simulink library "tqd"  (R2021b)
settings: Solver=VariableStepAuto  StartTime=0.0  StopTime=10.0  RelTol=1e-3
undefined symbols (not defined in the file or in its folder): ATQD_APSDecReq_X_kph, ATQD_APSDecReq_Y_mps2, ATQD_APSDecReqCMD_X_kph, ATQD_APSDecReqTs_X_pct, ATQD_APSDecTimeGain_X_Deg, ATQD_APSDecTimeGain_Y_s, ATQD_APSReqLowSpd_X_Deg, ATQD_AutoHoldReleaseBPS_X_Deg, ATQD_AWDLoadTrqnsGain_X_kg, ATQD_AWDLoadTrqnsGain_Y_pct, ATQD_BOSEnBPSPosn_X_kph, ATQD_BOSMap_X_rpm, ATQD_BOSMap_Y_pct, ATQD_CreepBaseTqD_X_kph, ATQD_CreepBaseTqD_Y_Deg, ATQD_CreepBaseTqR_X_kph, ATQD_CreepBaseTqR_Y_Deg, ATQD_CreepBPSDisPosn_X_Deg, ATQD_CreepBPSDisPosnR_X_Deg, ATQD_CreepBPSEnPosn_X_Deg, ATQD_CreepBPSEnPosnR_X_Deg, ATQD_CreepDeltaTq_X_kph, ATQD_CreepIterm_X_kph, ATQD_CreepIterm_Y_kph, ATQD_CreepItermMaxLimit_X_pct, ATQD_CreepPreloadTime_X_kph, ATQD_CreepPreloadTq_X_kph, ATQD_CreepPreloadTq_Y_s, ATQD_CreepProtTq_X_Deg, ATQD_CreepPterm_X_kph, ATQD_ECOTqMapD_X_rpm, ATQD_ECOTqMapD_Y_pct, ATQD_EOPDTqMapDCon_X_rpm, ATQD_EOPDTqMapDCon_Y_Deg, ATQD_EstInitVehWeight_X_c, ATQD_LHMRollGenMapD_X_rpm, ATQD_LHMRollGenMapD_Y_rpm, ATQD_LHMTqMapD_X_rpm, ATQD_LHMTqMapD_Y_pct, ATQD_NL1TqMapD_X_rpm, ATQD_NL1TqMapD_Y_pct, ATQD_NOPDTqMapDCon_X_rpm, ATQD_NOPDTqMapDCon_Y_Deg, ATQD_NRMRrEDUSpRat_X_rpm, ATQD_NRMRrEDUSpRat_Y_Nm, ATQD_OPDHoldDownRelDelay_X_Deg, ATQD_OPDHoldEnSpd_X_Deg, ATQD_OPDHoldRelDetTime_X_Deg, ATQD_OPDHoldReleaseTq_X_Deg, ATQD_OrigPedTqLowLim_X_Deg, ATQD_OrigPedTqLowLim_Y_pct, ATQD_PedalMapClimbUpLim_X_rpm, ATQD_PedalMapClimbUpLim_Y_Deg, ATQD_PreLoadTq_X_s, ATQD_RollGenMapEL1_X_rpm, ATQD_RollGenMapEL1_Y_rpm, ATQD_SL1TqMapD_X_rpm, ATQD_SL1TqMapD_Y_pct, ATQD_SlideRegenTqGain_X_Gps, ATQD_SlideRegenTqGain_Y_pct ... (+444)
libraries: hcu_lib x70, simulink x61, tqr x1
(part 8 of 14)

== system tqd/TQD/TorqueDemand/ShiftModule/GearShiftPosn/Drive Protection ==
  VINP_ShifterHandleCmd_enum : Inport
  VTQD_GearActualPosn_enum : Inport  Port=2
  VINP_VehSpeed_kph : Inport  Port=3
  VTQD_AfterAvailableTqDemFr_Nm : Inport  Port=4
  VTQR_NoABSREDUWhlTqReq_Nm : Inport  Port=5
  VTQR_NoABSFEDUWhlTqReq_Nm : Inport  Port=6
  VTQD_AfterAvailableTqDemRr_Nm : Inport  Port=7
  task_time_s : Inport  Port=8
  VTQD_BrkSwSta_flg : Inport  Port=9
  AND : Logic  Inputs=6  AllPortsSameDT=off  OutDataTypeStr=boolean
  AND1 : Logic  Commented=on  AllPortsSameDT=off  OutDataTypeStr=boolean
  AND2 : Logic  Inputs=3  AllPortsSameDT=off  OutDataTypeStr=boolean
  AND3 : Logic  Commented=on  Inputs=3  AllPortsSameDT=off  OutDataTypeStr=boolean
  AND4 : Logic  AllPortsSameDT=off  OutDataTypeStr=boolean
  Abs{,1,3..4} (4 alike) : Abs
  Add : Sum  Commented=on
  Add3 : Sum  Commented=on  Inputs=+++
  Constant1 : Constant  Commented=on  Value=ENUM_SHIFTCOMMAND_N
  Constant{3,6..7,10} (4 alike) : Constant  Value=KTQD_DrivProtEnToNTq_Nm
  Constant11 : Constant  Commented=on  Value=KTQD_CreepDisableSpdofst_kph
  Constant12 : Constant  Value=ENUM_SHIFTCOMMAND_N
  Constant13 : Constant  Value=KTQD_DriveProtVehSpdGain_kph
  Constant14 : Constant  Value=KTQD_DriveProtVehSpdGain_kph
  Constant16 : Constant  Value=KTQD_DrivProtEnSW_flg
  Constant17 : Constant  Value=KTQD_DriveProtDetTime_s
  Constant2 : Constant  Commented=on  Value=KTQD_DriveProtVehSpdGain_kph
  Constant20 : Constant  Commented=on  Value=ZERO_INT
  Constant21 : Constant  Commented=on  Value=ENUM_SHIFTCOMMAND_N
  Constant22 : Constant  Commented=on  Value=ENUM_SHIFTCOMMAND_N
  Constant23 : Constant  Commented=on  Value=ONE_INT
  Constant24 : Constant  Commented=on  Value=ZERO_INT
  Constant25 : Constant  Commented=on  Value=ENUM_SHIFTCOMMAND_NONE
  Constant26 : Constant  Commented=on  Value=KTQD_DriceProtDetTime_s
  Constant27 : Constant  Commented=on  Value=ENUM_SHIFTCOMMAND_D
  Constant29 : Constant  Commented=on  Value=ONE_INT
  Constant4 : Constant  Value=ENUM_GEARACTUALPOSN_D
  Constant5 : Constant  Commented=on  Value=ENUM_SHIFTCOMMAND_NONE
  Constant8 : Constant  Commented=on  Value=KTQD_DriveProtUpCount_c
  Constant9 : Constant  Commented=on  Value=KTQD_CreepEnableSpd_kph
  Delay : Delay  Commented=on  DelayLength=1
  Delay1 : Delay  Commented=on  DelayLength=1
  Delay2 : Delay  Commented=on  DelayLength=1
  Delay{4..8} (5 alike) : Delay  DelayLength=1
  DelayEnable : hcu_lib/Basic_Blocks/DelayEnable
  Detect Increase1 : simulink/Logic and Bit Operations/Detect Increase  Commented=on  vinit=0.0  OutDataTypeStr=boolean
  Equal{,2,6..7} (4 alike) : RelationalOperator  Operator=<=  OutDataTypeStr=boolean  RndMeth=Simplest
  Equal{1,4,12,15..16} (5 alike) : RelationalOperator  Commented=on  Operator===  OutDataTypeStr=boolean  RndMeth=Simplest
  Equal13 : RelationalOperator  Commented=on  Operator=~=  OutDataTypeStr=boolean  RndMeth=Simplest
  Equal14 : RelationalOperator  Commented=on  Operator=~=  OutDataTypeStr=boolean  RndMeth=Simplest
  Equal3 : RelationalOperator  Operator===  OutDataTypeStr=boolean  RndMeth=Simplest
  Equal5 : RelationalOperator  Commented=on  Operator=~=  OutDataTypeStr=boolean  RndMeth=Simplest
  Equal8 : RelationalOperator  Operator===  OutDataTypeStr=boolean  RndMeth=Simplest
  From1 : From  Commented=on  GotoTag=VINP_VehSpeed_kph
  From11 : From  Commented=on  GotoTag=VTQD_DriveProtCount_c
  From13 : From  Commented=on  GotoTag=VTQD_DriveProtDetFinish_flg
  From2 : From  Commented=on  GotoTag=VTQD_GearActualPosn_enum
  From32 : From  Commented=on  GotoTag=VTQD_DriveProtCount_c
  From{7,33..34,36} (4 alike) : From  Commented=on  GotoTag=VINP_ShifterHandleCmd_enum
  From35 : From  Commented=on  GotoTag=VTQD_DrivePortCountReset_flg
  From37 : From  Commented=on  GotoTag=VTQD_DriveProtDetFinish_flg
  From38 : From  Commented=on  GotoTag=VTQD_DriveProtDetFinish_flg
  From39 : From  Commented=on  GotoTag=task_time_s
  From40 : From  Commented=on  GotoTag=VTQD_GearActualPosn_enum
  Goto15 : Goto  Commented=on  GotoTag=VTQD_DrivePortCountReset_flg
  Goto16 : Goto  Commented=on  GotoTag=VTQD_DriveProtCount_c
  Goto17 : Goto  Commented=on  GotoTag=VTQD_DriveProtDetFinish_flg
  Goto9 : Goto  Commented=on  GotoTag=VTQD_DriveProtRemove_flg
  NOT : Logic  Commented=on  Operator=NOT  AllPortsSameDT=off  OutDataTypeStr=boolean
  NOT1 : Logic  Operator=NOT  AllPortsSameDT=off  OutDataTypeStr=boolean
  OR : Logic  Commented=on  Operator=OR  AllPortsSameDT=off  OutDataTypeStr=boolean
  OR1 : Logic  Operator=OR  AllPortsSameDT=off  OutDataTypeStr=boolean
  OR4 : Logic  Commented=on  Operator=OR  AllPortsSameDT=off  OutDataTypeStr=boolean
  OR5 : Logic  Commented=on  AllPortsSameDT=off  OutDataTypeStr=boolean
  Relational Operator1 : RelationalOperator  Commented=on  Operator=>  OutDataTypeStr=boolean  RndMeth=Simplest
  Relational Operator2 : RelationalOperator  Commented=on  OutDataTypeStr=boolean  RndMeth=Simplest
  Relational Operator3 : RelationalOperator  Operator=>  OutDataTypeStr=boolean  RndMeth=Simplest
  Relational Operator4 : RelationalOperator  Operator=<=  OutDataTypeStr=boolean  RndMeth=Simplest
  SR_Latch1 : hcu_lib/Basic_Blocks/SR_Latch  Commented=on
  SR_Latch2 : hcu_lib/Basic_Blocks/SR_Latch  Commented=on
  Switch10 : Switch  Commented=on  Criteria=u2 > Threshold
  Switch9 : Switch  Commented=on  Criteria=u2 > Threshold
  Timer : hcu_lib/Basic_Blocks/Timer  Commented=on
  VTQD_DriveProtRemove_flg : Outport
  VTQD_DriveProtToPsnN_flg : Outport  Port=2
  VTQD_DriveProtEn_flg : Outport  Port=3
  wires:
  [VTQD_DriveProtRemove_flg] -> AND/1
  Delay8/1 -> Equal3/1
  Abs4/1 -> Equal7/1
  Abs3/1 -> Equal6/1
  [VTQD_GearActualPosn_enum] -> Delay8/1
  Abs1/1 -> Equal2/1
  Abs/1 -> Equal/1
  AND2/1 -> VTQD_DriveProtEn_flg/1, DelayEnable/1  "VTQD_DriveProtEn_flg"
  Constant3/1 -> Equal/2
  Constant10/1 -> Equal2/2
  Constant6/1 -> Equal6/2
  Constant7/1 -> Equal7/2
  DelayEnable/1 -> [VTQD_DriveProtRemove_flg]  "VTQD_DriveProtRemove_flg"
  [task_time_s] -> DelayEnable/3
  Constant17/1 -> DelayEnable/2
  Constant16/1 -> AND2/2
  Equal8/1 -> AND2/1
  [VINP_VehSpeed_kph] -> Relational Operator3/1
  Constant14/1 -> Relational Operator3/2
  Constant12/1 -> Equal8/2
  [VINP_ShifterHandleCmd_enum] -> Equal8/1
  AND/1 -> [VTQD_DriveProtToPsnN_flg]  "VTQD_DriveProtToPsnN_flg"
  Delay7/1 -> [VTQD_AfterAvailableTqDemFr_Nm]
  Delay6/1 -> [VTQR_NoABSREDUWhlTqReq_Nm]
  Delay5/1 -> [VTQR_NoABSFEDUWhlTqReq_Nm]
  VTQR_NoABSFEDUWhlTqReq_Nm/1 -> Delay5/1
  Delay4/1 -> [VTQD_AfterAvailableTqDemRr_Nm]
  SR_Latch2/1 -> Goto9/1  "VTQD_DriveProtRemove_flg"
  task_time_s/1 -> [task_time_s]
  Constant2/1 -> Add3/1
  Constant11/1 -> Add3/3
  Add3/1 -> Relational Operator1/2
  Constant9/1 -> Add3/2
  VTQD_AfterAvailableTqDemRr_Nm/1 -> Delay4/1
  Equal7/1 -> AND/6
  [VTQD_AfterAvailableTqDemFr_Nm] -> Abs4/1
  Equal6/1 -> AND/5
  [VTQR_NoABSFEDUWhlTqReq_Nm] -> Abs3/1
  [VTQD_DriveProtToPsnN_flg] -> VTQD_DriveProtToPsnN_flg/1
  VTQR_NoABSREDUWhlTqReq_Nm/1 -> Delay6/1
  VTQD_AfterAvailableTqDemFr_Nm/1 -> Delay7/1
  VINP_VehSpeed_kph/1 -> [VINP_VehSpeed_kph]
  VTQD_GearActualPosn_enum/1 -> [VTQD_GearActualPosn_enum]
  VINP_ShifterHandleCmd_enum/1 -> [VINP_ShifterHandleCmd_enum]
  OR/1 -> SR_Latch2/2
  Equal5/1 -> OR/2
  Equal1/1 -> OR/1
  Constant5/1 -> Equal5/2
  From7/1 -> Equal5/1
  Constant4/1 -> Equal3/2
  Equal3/1 -> AND/4
  [VTQR_NoABSREDUWhlTqReq_Nm] -> Abs1/1
  Equal2/1 -> AND/3
  Equal/1 -> AND/2
  [VTQD_AfterAvailableTqDemRr_Nm] -> Abs/1
  [VTQD_DriveProtRemove_flg] -> VTQD_DriveProtRemove_flg/1
  Constant1/1 -> Equal1/2
  From2/1 -> Equal1/1
  Relational Operator1/1 -> AND3/3
  From1/1 -> Relational Operator1/1
  From11/1 -> Equal4/1
  From13/1 -> AND1/2
  Constant8/1 -> Equal4/2
  AND1/1 -> SR_Latch2/1  "VTQD_DriveProtEn_flg"
  Equal4/1 -> AND1/1
  Delay2/1 -> SR_Latch1/2
  Equal13/1 -> OR5/1
  Switch9/1 -> Add/1
  Switch10/1 -> Delay/1
  Constant24/1 -> Switch10/1
  From35/1 -> Switch10/2
  Detect Increase1/1 -> Switch9/2  "VTQD_ShiftNRiseDet_flg"
  From36/1 -> Equal12/1
  OR4/1 -> Goto15/1  "VTQD_DrivePortCountReset_flg"
  Equal14/1 -> OR5/2
  Add/1 -> Switch10/3
  From33/1 -> Equal13/1
  Constant29/1 -> Equal16/2
  Constant22/1 -> Equal13/2
  Delay/1 -> Add/2, Goto16/1  "VTQD_DriveProtCount_c"
  Equal15/1 -> AND3/2
  From34/1 -> Equal14/1
  Relational Operator2/1 -> Goto17/1  "VTQD_DriveProtDetFinish_flg"
  Constant20/1 -> Switch9/3
  Timer/1 -> Relational Operator2/1  "VTQD_DriveProtDetTime_s"
  OR5/1 -> OR4/2
  AND3/1 -> SR_Latch1/1  "VTQD_DriveProtTimerEn_flg"
  NOT/1 -> Timer/2
  Constant21/1 -> Equal12/2
  Constant25/1 -> Equal14/2
  From39/1 -> Timer/3
  From32/1 -> Equal16/1
  From37/1 -> Delay1/1
  From40/1 -> Equal15/1
  From38/1 -> Delay2/1
  Delay1/1 -> OR4/1
  SR_Latch1/1 -> Timer/1, NOT/1
  Constant27/1 -> Equal15/2
  Constant23/1 -> Switch9/1
  Equal16/1 -> AND3/1
  Equal12/1 -> Detect Increase1/1
  Constant26/1 -> Timer/4, Relational Operator2/2
  OR1/1 -> AND2/3
  Relational Operator3/1 -> OR1/1
  Constant13/1 -> Relational Operator4/2
  [VINP_VehSpeed_kph] -> Relational Operator4/1
  Relational Operator4/1 -> AND4/1
  AND4/1 -> OR1/2
  [VTQD_BrkSwSta_flg] -> NOT1/1
  NOT1/1 -> AND4/2
  VTQD_BrkSwSta_flg/1 -> [VTQD_BrkSwSta_flg]

== system tqd/TQD/TorqueDemand/Signal_convert/Regen Level Switch Botton/RegenDOWN ==
  note: IF PRESS BOTH then nothing happen
  note: Long press or Short press
  note: If press time more then Long press's limit then go Long press only. Else go short press only. Else if no press.
  note: IF PRESS BOTH then nothing happen
  task_time_s : Inport
  SWC_RegenUp : Inport  Port=2
  SWC_RegenDOWN : Inport  Port=3
  AND : Logic  AllPortsSameDT=off  OutDataTypeStr=boolean
  AND1 : Logic  AllPortsSameDT=off  OutDataTypeStr=boolean
  AND2 : Logic  AllPortsSameDT=off  OutDataTypeStr=boolean
  Constant{1..2,4,7,10} (5 alike) : Constant  Value=FALSE
  Constant3 : Constant  Value=KTQD_RegShortPLim_s
  Default 3 sec : Constant  Value=KTQD_RegLongPLim_s
  DelayEnable_LONG_PRESS : hcu_lib/Basic_Blocks/DelayEnable
  DelayEnable_SHORT_PRESS : hcu_lib/Basic_Blocks/DelayEnable
  Detect Decrease1 : simulink/Logic and Bit Operations/Detect Decrease  vinit=0.0  OutDataTypeStr=boolean
  Detect Decrease2 : simulink/Logic and Bit Operations/Detect Decrease  vinit=0.0  OutDataTypeStr=boolean
  Detect Increase : simulink/Logic and Bit Operations/Detect Increase  vinit=0.0  OutDataTypeStr=boolean
  NOT : Logic  Operator=NOT  AllPortsSameDT=off  OutDataTypeStr=boolean
  NOT1 : Logic  Operator=NOT  AllPortsSameDT=off  OutDataTypeStr=boolean
  SR_Latch : hcu_lib/Basic_Blocks/SR_Latch
  Switch{1..5} (5 alike) : Switch  Criteria=u2 ~= 0
  SWC_RegenDownShort_flg : Outport
  VTQD_RegenDownLongP_flg : Outport  Port=2
  wires:
  Detect Decrease1/1 -> AND/2
  SR_Latch/1 -> [PRESS_BOTH]
  AND2/1 -> SR_Latch/2
  NOT1/1 -> AND2/2
  NOT/1 -> AND2/1
  [SWC_RegenDOWN] -> NOT1/1
  [SWC_RegenUp] -> NOT/1
  Constant4/1 -> Switch5/1
  [PRESS_BOTH] -> Switch5/2
  [SWC_RegenDOWN] -> Switch5/3
  Switch4/1 -> [Short_press_falling_Edge]
  Detect Decrease2/1 -> Switch4/3
  [PRESS_BOTH] -> Switch4/2
  Constant2/1 -> Switch4/1
  Constant1/1 -> Switch3/1
  AND1/1 -> SR_Latch/1
  [SWC_RegenUp] -> AND1/1
  [SWC_RegenDOWN] -> AND1/2
  [PRESS_BOTH] -> Switch3/2
  SWC_RegenDOWN/1 -> [SWC_RegenDOWN]
  SWC_RegenUp/1 -> [SWC_RegenUp]
  Switch3/1 -> [Long_press]
  Switch2/1 -> SWC_RegenDownShort_flg/1
  AND/1 -> Switch2/2
  Switch5/1 -> DelayEnable_LONG_PRESS/1, DelayEnable_SHORT_PRESS/1
  [Short_press_falling_Edge] -> Switch2/3
  Constant10/1 -> Switch2/1
  [Long_press] -> Detect Increase/1, Detect Decrease1/1
  [Short_press_falling_Edge] -> AND/1
  Switch1/1 -> Switch3/3
  DelayEnable_LONG_PRESS/1 -> Switch1/2, Switch1/1
  Constant7/1 -> Switch1/3
  DelayEnable_SHORT_PRESS/1 -> Detect Decrease2/1
  Constant3/1 -> DelayEnable_SHORT_PRESS/2
  [task_time_s] -> DelayEnable_SHORT_PRESS/3
  Default 3 sec/1 -> DelayEnable_LONG_PRESS/2
  [task_time_s] -> DelayEnable_LONG_PRESS/3
  Detect Increase/1 -> VTQD_RegenDownLongP_flg/1
  task_time_s/1 -> [task_time_s]

== system tqd/TQD/TorqueDemand/Signal_convert/Regen Level Switch Botton/RegenUP ==
  note: IF PRESS BOTH then nothing happen
  note: Long press or Short press
  note: If press time more then Long press's limit then go Long press only. Else go short press only. Else if no press.
  note: IF PRESS BOTH then nothing happen
  task_time_s : Inport
  SWC_RegenUp : Inport  Port=2
  SWC_RegenDOWN : Inport  Port=3
  AND : Logic  AllPortsSameDT=off  OutDataTypeStr=boolean
  AND1 : Logic  AllPortsSameDT=off  OutDataTypeStr=boolean
  AND2 : Logic  AllPortsSameDT=off  OutDataTypeStr=boolean
  Constant{1..2,4,7,10} (5 alike) : Constant  Value=FALSE
  Constant3 : Constant  Value=KTQD_RegShortPLim_s
  Default 3 sec : Constant  Value=KTQD_RegLongPLim_s
  DelayEnable_LONG_PRESS : hcu_lib/Basic_Blocks/DelayEnable
  DelayEnable_SHORT_PRESS : hcu_lib/Basic_Blocks/DelayEnable
  Detect Decrease1 : simulink/Logic and Bit Operations/Detect Decrease  vinit=0.0  OutDataTypeStr=boolean
  Detect Decrease2 : simulink/Logic and Bit Operations/Detect Decrease  vinit=0.0  OutDataTypeStr=boolean
  Detect Increase : simulink/Logic and Bit Operations/Detect Increase  vinit=0.0  OutDataTypeStr=boolean
  NOT : Logic  Operator=NOT  AllPortsSameDT=off  OutDataTypeStr=boolean
  NOT1 : Logic  Operator=NOT  AllPortsSameDT=off  OutDataTypeStr=boolean
  SR_Latch : hcu_lib/Basic_Blocks/SR_Latch
  Switch{1..5} (5 alike) : Switch  Criteria=u2 ~= 0
  SWC_RegenUpShort_flg : Outport
  VTQD_RegenUpLongP_flg : Outport  Port=2
  wires:
  Detect Decrease1/1 -> AND/2
  SR_Latch/1 -> [PRESS_BOTH]
  AND2/1 -> SR_Latch/2
  NOT1/1 -> AND2/2
  NOT/1 -> AND2/1
  [SWC_RegenDOWN] -> NOT1/1
  [SWC_RegenUp] -> NOT/1
  Constant4/1 -> Switch5/1
  [PRESS_BOTH] -> Switch5/2
  [SWC_RegenUp] -> Switch5/3
  Switch4/1 -> [Short_press_falling_Edge]
  Detect Decrease2/1 -> Switch4/3
  [PRESS_BOTH] -> Switch4/2
  Constant2/1 -> Switch4/1
  Constant1/1 -> Switch3/1
  AND1/1 -> SR_Latch/1
  [SWC_RegenUp] -> AND1/1
  [SWC_RegenDOWN] -> AND1/2
  [PRESS_BOTH] -> Switch3/2
  SWC_RegenDOWN/1 -> [SWC_RegenDOWN]
  SWC_RegenUp/1 -> [SWC_RegenUp]
  Switch3/1 -> [Long_press]
  Switch2/1 -> SWC_RegenUpShort_flg/1
  AND/1 -> Switch2/2
  Switch5/1 -> DelayEnable_LONG_PRESS/1, DelayEnable_SHORT_PRESS/1
  [Short_press_falling_Edge] -> Switch2/3
  Constant10/1 -> Switch2/1
  [Long_press] -> Detect Increase/1, Detect Decrease1/1
  [Short_press_falling_Edge] -> AND/1
  Switch1/1 -> Switch3/3
  DelayEnable_LONG_PRESS/1 -> Switch1/2, Switch1/1
  Constant7/1 -> Switch1/3
  DelayEnable_SHORT_PRESS/1 -> Detect Decrease2/1
  Constant3/1 -> DelayEnable_SHORT_PRESS/2
  [task_time_s] -> DelayEnable_SHORT_PRESS/3
  Default 3 sec/1 -> DelayEnable_LONG_PRESS/2
  [task_time_s] -> DelayEnable_LONG_PRESS/3
  Detect Increase/1 -> VTQD_RegenUpLongP_flg/1
  task_time_s/1 -> [task_time_s]

== system tqd/TQD/TorqueDemand/Signal_convert/Speed Setting Mode/ACC Speed Setting ON ==
  note: ACC SPEED SETTING MODE
  VTQD_SWCResUpSta_flg : Inport
  VTQD_SWCSetDownSta_flg : Inport  Port=2
  task_time_s : Inport  Port=3
  VVMC_LVDAACCStatusInformation_flg : Inport  Port=4
  VVMC_ACCObjDist_m : Inport  Port=5
  VVMC_MeterIndSpeed_raw32 : Inport  Port=6
  VINP_ADASACCSta_enum : Inport  Port=7
  VINP_Distanceunit_flg : Inport  Port=8
  Action Port : ActionPort  InitializeStates=reset
  " 20" : Constant  Value=KTQD_ACCActiveMetSpdLoMPH_mph
  " 30kph" : Constant  Value=KTQD_ACCActiveMetSpdLo_kph
  0 : Constant  Value=KTQD_AllowSetSpdOvrd_flg
  1 : Constant  Value=KTQD_AllowSetSpdOvrdVal_flg
  1.1s : Constant  Value=KTQD_SetSpdLongPLim_s
  105 : Constant  Value=KTQD_ACCActiveMetSpdHiMPH_mph
  10kph1 : Constant  Value=KTQD_AllowSetSpdSpd_kph
  180kph : Constant  Value=KTQD_ACCActiveMetSpdHi_kph
  20m : Constant  Value=KTQD_AllowSetSpdDist_m
  2m : Constant  Value=KTQD_NotAllowSetSpdDist_m
  5 : Constant  Value=KTQD_SetSpdDeltaLongMPH_mph
  5kph : Constant  Value=KTQD_SetSpdDeltaLong_kph
  ACCSetSpd_Chart_W : Stateflow chart  TreatAsAtomicUnit=on
      settings: PortSchema="{\"entries\":[{\"content\":{\"sides\":[{\"content\":{\"connectorIds\":[\"In1\",\"In2\",\"In3\",\"In4\",\"In5\",\"In6\",\"In7\",\"In8\",\"In12\",\"In9\",\"In10\",\"In11\"]},\"type\":\"ConnectorPlacement.EquallySpacedRectSide\",\"uuid\":\"61ce72b2-2f56-4065-9e06-1345412a8c86\"},{\"content\":{\"connectorIds\":[\"Out1\"],\"side\":\"RIGHT\"},\"type\":\"ConnectorPlacement.EquallySpacedRectSide\",\"uuid\":\"4594d6d3-f7cd-4711-8df0-9a0a2c5601b5\"},{\"content\":{\"connectorIds\":[],\"side\":\"TOP\"},\"type\":\"ConnectorPlacement.EquallySpacedRectSide\",\"uuid\":\"a8857ab2-f9b0-4737-b2f3-522f42c1ada3\"}]},\"type\":\"ConnectorPlacement.EquallySpacedConnector\",\"uuid\":\"0a7f8e6a-9c19-454d-bd26-d3d8923cc49e\"}],\"packageUris\":[\"http://schema.mathworks.com/mf0/Connector/R2020b\"],\"version\":\"1.0\"}"
  AND : Logic  AllPortsSameDT=off  OutDataTypeStr=boolean
  AND1 : Logic  AllPortsSameDT=off  OutDataTypeStr=boolean
  Cast To Single : DataTypeConversion  OutDataTypeStr=int8
  ONE : Constant  Value=ONE_INT
  OR : Logic  Operator=OR  AllPortsSameDT=off  OutDataTypeStr=boolean
  Relational Operator : RelationalOperator  Operator=<=  OutDataTypeStr=boolean  RndMeth=Simplest
  Relational Operator1 : RelationalOperator  Operator=>  OutDataTypeStr=boolean  RndMeth=Simplest
  Relational Operator2 : RelationalOperator  Operator===  OutDataTypeStr=boolean  RndMeth=Simplest
  Relational Operator3 : RelationalOperator  OutDataTypeStr=boolean  RndMeth=Simplest
  Relational Operator4 : RelationalOperator  Operator===  OutDataTypeStr=boolean  RndMeth=Simplest
  Round : Rounding  Operator=round
  Switch{,1..4} (5 alike) : Switch  Criteria=u2 > Threshold
  standby : Constant  Value=ENUM_ADASACCSTA_STANDBY
  zero : Constant  Value=ZERO_INT
  VTQD_ACCSetSpd_kph : Outport
  wires:
  VVMC_LVDAACCStatusInformation_flg/1 -> ACCSetSpd_Chart_W/10(VVMC_LVDAACCStatusInformation_flg)
  1.1s/1 -> ACCSetSpd_Chart_W/9(KTQD_SetSpdLongPLim_s)
  task_time_s/1 -> ACCSetSpd_Chart_W/12(task_time_s)
  Switch4/1 -> ACCSetSpd_Chart_W/8(KTQD_SetSpdDeltaLong_kph)
  Switch3/1 -> ACCSetSpd_Chart_W/7(KTQD_ACCActiveMetSpdLo_raw32)
  180kph/1 -> Switch2/3
  VVMC_MeterIndSpeed_raw32/1 -> ACCSetSpd_Chart_W/4(VVMC_MeterIndSpeed_raw32), [VVMC_MeterIndSpeed_raw32]
  VTQD_SWCSetDownSta_flg/1 -> ACCSetSpd_Chart_W/3(VTQD_SWCSetDownSta_flg)
  VTQD_SWCResUpSta_flg/1 -> ACCSetSpd_Chart_W/2(VTQD_SWCResUpSta_flg)
  VINP_ADASACCSta_enum/1 -> [VINP_ADASACCSta_enum], ACCSetSpd_Chart_W/1(VINP_ADASACCSta_enum)
  VVMC_ACCObjDist_m/1 -> Relational Operator/1, Relational Operator1/1
  20m/1 -> Relational Operator/2
  2m/1 -> Relational Operator1/2
  Relational Operator/1 -> AND/1
  Relational Operator1/1 -> AND/2
  [VVMC_MeterIndSpeed_raw32] -> Relational Operator3/1
  10kph1/1 -> Relational Operator3/2
  AND/1 -> OR/1
  Relational Operator3/1 -> OR/2
  Switch/1 -> [VTQD_AllowSetSpd_flg]
  OR/1 -> Switch/3
  0/1 -> Switch/2
  1/1 -> Switch/1
  [VTQD_AllowSetSpd_flg] -> ACCSetSpd_Chart_W/11(VTQD_AllowSetSpd_flg)
  Cast To Single/1 -> Relational Operator4/1, Switch1/3
  Switch1/1 -> VTQD_ACCSetSpd_kph/1
  [VINP_ADASACCSta_enum] -> Relational Operator2/1
  AND1/1 -> Switch1/2
  ONE/1 -> Switch1/1
  standby/1 -> Relational Operator2/2
  zero/1 -> Relational Operator4/2
  Relational Operator2/1 -> AND1/1
  Relational Operator4/1 -> AND1/2
  VINP_Distanceunit_flg/1 -> [VINP_Distanceunit_flg]
  [VINP_Distanceunit_flg] -> Switch2/2
  105/1 -> Switch2/1
  Switch2/1 -> ACCSetSpd_Chart_W/5(KTQD_ACCActiveMetSpdHi_raw32)
  [VINP_Distanceunit_flg] -> Switch3/2
  " 30kph"/1 -> Switch3/3
  " 20"/1 -> Switch3/1
  [VINP_Distanceunit_flg] -> Switch4/2
  5kph/1 -> Switch4/3
  5/1 -> Switch4/1
  [VINP_Distanceunit_flg] -> ACCSetSpd_Chart_W/6(VINP_Distanceunit_flg)
  Round/1 -> Cast To Single/1
  ACCSetSpd_Chart_W/1(VTQD_ACCSetSpd_kph) -> Round/1

== system tqd/TQD/TorqueDemand/Signal_convert/Speed Setting Mode/CC Speed Setting ON ==
  note: CC SPEED SETTING MODE
  VVMC_CCCtrlSta_enum : Inport
  "VTQD_SWCResUpPress_enum  " : Inport  Port=2
  "VTQD_SWCSetDownPress_enum  " : Inport  Port=3
  VVMC_MeterIndSpeed_raw32 : Inport  Port=4
  VTQD_SetSpdDeltaLongFit_kph : Inport  Port=5
  VINP_Distanceunit_flg : Inport  Port=6
  Action Port : ActionPort  InitializeStates=reset
  " 1" : Constant  Value=KTQD_CCActiveMetSpdLo_kph
  " 2" : Constant  Value=KTQD_CCActiveMetSpdLoMPH_mph
  1 : Constant  Value=KTQD_SetSpdDeltaLongFit_kph
  2 : Constant  Value=KTQD_SetSpdDeltaShort_kph
  3 : Constant  Value=KTQD_CCActiveMetSpdHi_kph
  4 : Constant  Value=KTQD_SetSpdDeltaLong_kph
  5 : Constant  Value=KTQD_CCActiveMetSpdHiMPH_mph
  6 : Constant  Value=KTQD_SetSpdDeltaLongMPH_mph
  AND1 : Logic  AllPortsSameDT=off  OutDataTypeStr=boolean
  CC Speed Setting Mode : Stateflow chart  TreatAsAtomicUnit=on
      settings: PortSchema="{\"entries\":[{\"content\":{\"sides\":[{\"content\":{\"connectorIds\":[\"In5\",\"In12\",\"In4\",\"In3\",\"In9\",\"In6\",\"In7\",\"In8\",\"In1\",\"In2\",\"In11\",\"In10\"]},\"type\":\"ConnectorPlacement.EquallySpacedRectSide\",\"uuid\":\"331c8dfa-4564-419d-9323-fdbf8561d50b\"},{\"content\":{\"connectorIds\":[\"Out1\",\"Out2\"],\"side\":\"RIGHT\"},\"type\":\"ConnectorPlacement.EquallySpacedRectSide\",\"uuid\":\"71cb1444-7708-4b6f-91dd-d8a1c8c14ea8\"},{\"content\":{\"connectorIds\":[],\"side\":\"TOP\"},\"type\":\"ConnectorPlacement.EquallySpacedRectSide\",\"uuid\":\"6ecf38bb-d171-491a-a8b2-073f135e7039\"}]},\"type\":\"ConnectorPlacement.EquallySpacedConnector\",\"uuid\":\"fc3afa97-6e6e-4933-9aff-7c8f8cbb1702\"}],\"packageUris\":[\"http://schema.mathworks.com/mf0/Connector/R2020b\"],\"version\":\"1.0\"}"
  Cast To Single : DataTypeConversion  OutDataTypeStr=int8
  ONE : Constant  Value=ONE_INT
  Relational Operator2 : RelationalOperator  Operator===  OutDataTypeStr=boolean  RndMeth=Simplest
  Relational Operator4 : RelationalOperator  Operator===  OutDataTypeStr=boolean  RndMeth=Simplest
  Round : Rounding  Operator=round
  Specific_STATE_ChangeToSTANDBY : Stateflow chart  TreatAsAtomicUnit=on
  Switch{1..4} (4 alike) : Switch  Criteria=u2 > Threshold
  Terminator1 : Terminator
  standby : Constant  Value=ENUM_ADASCCSTA_STANDBY
  zero : Constant  Value=ZERO_INT
  VTQD_CCSetSpd_kph : Outport
  wires:
  "VTQD_SWCSetDownPress_enum  "/1 -> CC Speed Setting Mode/10(VTQD_SWCSetDownPress_enum)
  [VTQD_ChangeToSTANDBY_flg] -> CC Speed Setting Mode/12(VTQD_ChangeToSTANDBY_flg)
  Specific_STATE_ChangeToSTANDBY/1(VTQD_CCChangeToSTANDBY_flg) -> [VTQD_ChangeToSTANDBY_flg]  "VTQD_CCChangeToSTANDBY_flg"
  [VVMC_CCCtrlSta_enum] -> Specific_STATE_ChangeToSTANDBY/1(VVMC_CCCtrlSta_enum)
  "VTQD_SWCResUpPress_enum  "/1 -> CC Speed Setting Mode/11(VTQD_SWCResUpPress_enum)
  VVMC_CCCtrlSta_enum/1 -> CC Speed Setting Mode/5(VVMC_CCCtrlSta_enum), [VVMC_CCCtrlSta_enum]
  Switch2/1 -> CC Speed Setting Mode/7(KTQD_CCActiveMetSpdHi_raw32)
  2/1 -> CC Speed Setting Mode/2(KTQD_SetSpdDeltaShort_kph)
  Switch3/1 -> CC Speed Setting Mode/8(KTQD_CCActiveMetSpdLo_raw32)
  Switch4/1 -> CC Speed Setting Mode/1(KTQD_SetSpdDeltaLong_kph)
  CC Speed Setting Mode/2(VTQD_CCSpdResetFinish_flg) -> Terminator1/1  "VTQD_CCSpdResetFinish_flg"
  VTQD_SetSpdDeltaLongFit_kph/1 -> CC Speed Setting Mode/4(VTQD_SetSpdDeltaLongFit_kph)
  1/1 -> CC Speed Setting Mode/3(KTQD_SetSpdDeltaLongFit_kph)
  VVMC_MeterIndSpeed_raw32/1 -> CC Speed Setting Mode/9(VVMC_MeterIndSpeed_raw32)
  Cast To Single/1 -> Relational Operator4/1, Switch1/3
  Switch1/1 -> VTQD_CCSetSpd_kph/1
  [VVMC_CCCtrlSta_enum] -> Relational Operator2/1
  AND1/1 -> Switch1/2
  ONE/1 -> Switch1/1
  standby/1 -> Relational Operator2/2
  zero/1 -> Relational Operator4/2
  Relational Operator2/1 -> AND1/1
  Relational Operator4/1 -> AND1/2
  [VINP_Distanceunit_flg] -> Switch2/2
  VINP_Distanceunit_flg/1 -> [VINP_Distanceunit_flg]
  3/1 -> Switch2/3
  5/1 -> Switch2/1
  [VINP_Distanceunit_flg] -> Switch3/2
  " 1"/1 -> Switch3/3
  " 2"/1 -> Switch3/1
  [VINP_Distanceunit_flg] -> Switch4/2
  4/1 -> Switch4/3
  6/1 -> Switch4/1
  [VINP_Distanceunit_flg] -> CC Speed Setting Mode/6(VINP_Distanceunit_flg)
  Round/1 -> Cast To Single/1
  CC Speed Setting Mode/1(VTQD_CCSetSpd_kph) -> Round/1

== system tqd/TQD/TorqueDemand/Signal_convert/Speed Setting Mode/Else Speed Setting On ==
  In : Inport
  Action Port : ActionPort
  Data Type Conversion : DataTypeConversion
  Out : Outport
  wires:
  Data Type Conversion/1 -> Out/1
  In/1 -> Data Type Conversion/1

== system tqd/TQD/TorqueDemand/Signal_convert/Speed Setting Mode/ISA Speed Setting ON ==
  VINP_ADASVehSpdLim_kph : Inport
  Action Port : ActionPort
  Data Type Conversion : DataTypeConversion
  VTQD_ISASetSpd_kph : Outport
  wires:
  VINP_ADASVehSpdLim_kph/1 -> Data Type Conversion/1
  Data Type Conversion/1 -> VTQD_ISASetSpd_kph/1

== system tqd/TQD/TorqueDemand/Signal_convert/Speed Setting Mode/MSA Speed Setting ON ==
  note: MSA SPEED SETTING MODE
  VVMC_MSACrlSta_enum : Inport
  "VTQD_SWCResUpPress_enum  " : Inport  Port=2
  "VTQD_SWCSetDownPress_enum  " : Inport  Port=3
  VVMC_MeterIndSpeed_raw32 : Inport  Port=4
  VTQD_SetSpdDeltaLongFit_kph : Inport  Port=5
  VINP_Distanceunit_flg : Inport  Port=6
  Action Port : ActionPort  InitializeStates=reset
  " 1" : Constant  Value=KTQD_MSAActiveMetSpdLoMPH_mph
  " 80" : Constant  Value=KTQD_MSAActiveMetSpdLo_kph
  1 : Constant  Value=KTQD_SetSpdDeltaShort_kph
  160 : Constant  Value=KTQD_MSAActiveMetSpdHi_kph
  2 : Constant  Value=KTQD_MSAActiveMetSpdHiMPH_mph
  3 : Constant  Value=KTQD_SetSpdDeltaLongMPH_mph
  5 : Constant  Value=KTQD_SetSpdDeltaLong_kph
  AND1 : Logic  AllPortsSameDT=off  OutDataTypeStr=boolean
  Cast To Single : DataTypeConversion  OutDataTypeStr=int8
  Delta Long Fit Base : Constant  Value=KTQD_SetSpdDeltaLongFit_kph
  MSA : Stateflow chart  TreatAsAtomicUnit=on
      settings: PortSchema="{\"entries\":[{\"content\":{\"sides\":[{\"content\":{\"connectorIds\":[\"In9\",\"In6\",\"In5\",\"In4\",\"In7\",\"In8\",\"In1\",\"In2\",\"In12\",\"In10\",\"In11\",\"In3\"]},\"type\":\"ConnectorPlacement.EquallySpacedRectSide\",\"uuid\":\"4fee65fe-2e32-4dfc-9c8c-ef7087e97952\"},{\"content\":{\"connectorIds\":[\"Out1\"],\"side\":\"RIGHT\"},\"type\":\"ConnectorPlacement.EquallySpacedRectSide\",\"uuid\":\"8d915692-cb0b-4a06-a57e-690cea51e532\"},{\"content\":{\"connectorIds\":[],\"side\":\"TOP\"},\"type\":\"ConnectorPlacement.EquallySpacedRectSide\",\"uuid\":\"3fa43362-4ddf-4693-9d82-d4f790f00c9c\"}]},\"type\":\"ConnectorPlacement.EquallySpacedConnector\",\"uuid\":\"c1a6cfdc-58f2-45b0-af62-575976a00cf2\"}],\"packageUris\":[\"http://schema.mathworks.com/mf0/Connector/R2020b\"],\"version\":\"1.0\"}"
  ONE : Constant  Value=ONE_INT
  Relational Operator2 : RelationalOperator  Operator===  OutDataTypeStr=boolean  RndMeth=Simplest
  Relational Operator4 : RelationalOperator  Operator===  OutDataTypeStr=boolean  RndMeth=Simplest
  Round : Rounding  Operator=round
  Specific_STATE_ChangeToOFF : Stateflow chart  TreatAsAtomicUnit=on
  Switch{1..4} (4 alike) : Switch  Criteria=u2 > Threshold
  standby : Constant  Value=ENUM_ADASMSASTA_STANDBY
  zero : Constant  Value=ZERO_INT
  VSCP_MSASetSpd_kph : Outport
  wires:
  VVMC_MeterIndSpeed_raw32/1 -> MSA/6(VVMC_MeterIndSpeed_raw32)
  Delta Long Fit Base/1 -> MSA/11(KTQD_SetSpdDeltaLongFit_kph)
  VTQD_SetSpdDeltaLongFit_kph/1 -> MSA/10(VTQD_SetSpdDeltaLongFit_kph)
  Switch2/1 -> MSA/7(KTQD_MSAActiveMetSpdHi_raw32)
  Switch3/1 -> MSA/8(KTQD_MSAActiveMetSpdLo_raw32)
  VVMC_MSACrlSta_enum/1 -> [VINP_MSACrlSta_enum], MSA/9(VVMC_MSACrlSta_enum)
  1/1 -> MSA/2(KTQD_SetSpdDeltaShort_kph)
  Switch4/1 -> MSA/1(KTQD_SetSpdDeltaLong_kph)
  [VTQD_ChangeToOFF_flg] -> MSA/5(VTQD_ChangeToOFF_flg)
  "VTQD_SWCSetDownPress_enum  "/1 -> MSA/3(VTQD_SWCSetDownPress_enum)
  "VTQD_SWCResUpPress_enum  "/1 -> MSA/12(VTQD_SWCResUpPress_enum)
  Specific_STATE_ChangeToOFF/1(VTQD_ChangeToOFF_flg) -> [VTQD_ChangeToOFF_flg]  "VTQD_ChangeToOFF_flg"
  [VINP_MSACrlSta_enum] -> Specific_STATE_ChangeToOFF/1(VINP_MSACrlSta_enum)
  AND1/1 -> Switch1/2
  zero/1 -> Relational Operator4/2
  standby/1 -> Relational Operator2/2
  ONE/1 -> Switch1/1
  Cast To Single/1 -> Relational Operator4/1, Switch1/3
  Relational Operator2/1 -> AND1/1
  [VINP_MSACrlSta_enum] -> Relational Operator2/1
  Relational Operator4/1 -> AND1/2
  Switch1/1 -> VSCP_MSASetSpd_kph/1
  [VINP_Distanceunit_flg] -> Switch2/2
  VINP_Distanceunit_flg/1 -> [VINP_Distanceunit_flg]
  160/1 -> Switch2/3
  2/1 -> Switch2/1
  [VINP_Distanceunit_flg] -> Switch3/2
  " 80"/1 -> Switch3/3
  " 1"/1 -> Switch3/1
  [VINP_Distanceunit_flg] -> Switch4/2
  5/1 -> Switch4/3
  3/1 -> Switch4/1
  [VINP_Distanceunit_flg] -> MSA/4(VINP_Distanceunit_flg)
  Round/1 -> Cast To Single/1
  MSA/1(VTQD_MSASetSpd_kph) -> Round/1

== system tqd/TQD/TorqueDemand/Signal_convert/Speed Setting Mode/VTQD_SWCCancelP_flg ==
  INPUT : Inport
  Detect Decrease : simulink/Logic and Bit Operations/Detect Decrease  vinit=0.0  OutDataTypeStr=boolean
  Falling_edge : Outport
  wires:
  Detect Decrease/1 -> Falling_edge/1
  INPUT/1 -> Detect Decrease/1

== system tqd/TQD/TorqueDemand/Signal_convert/Speed Setting Mode/VTQD_SWCResUpPress_enum ==
  note: Long press or Short press
  INPUT : Inport
  task_time_s : Inport  Port=2
  AND : Logic  AllPortsSameDT=off  OutDataTypeStr=boolean
  AND1 : Logic  AllPortsSameDT=off  OutDataTypeStr=boolean
  Constant2 : Constant  Value=KTQD_SetSpdShortPLim_s
  Constant3 : Constant  Value=KTQD_SetSpdLongPLim_s
  Constant4 : Constant  Value=ENUM_SWCBOTTONPRESS_LONGPRESS
  Constant5 : Constant  Value=ENUM_SWCBOTTONPRESS_SHORTPRESS
  Constant6 : Constant  Value=ENUM_SWCBOTTONPRESS_NOPRESS
  Delay : Delay  DelayLength=1
  DelayEnable_LONG_PRESS1 : hcu_lib/Basic_Blocks/DelayEnable
  DelayEnable_SHORT_PRESS1 : hcu_lib/Basic_Blocks/DelayEnable
  Detect Decrease : simulink/Logic and Bit Operations/Detect Decrease  vinit=0.0  OutDataTypeStr=boolean
  Detect Decrease4 : simulink/Logic and Bit Operations/Detect Decrease  vinit=0.0  OutDataTypeStr=boolean
  NOT : Logic  Operator=NOT  AllPortsSameDT=off  OutDataTypeStr=boolean
  NOT1 : Logic  Operator=NOT  AllPortsSameDT=off  OutDataTypeStr=boolean
  SR_Latch : hcu_lib/Basic_Blocks/SR_Latch
  Switch : Switch  Criteria=u2 ~= 0
  Switch3 : Switch  Criteria=u2 ~= 0
  OUTPUT : Outport
  wires:
  [Short_press_falling_Edge] -> Switch3/2
  Detect Decrease/1 -> SR_Latch/2
  [INPUT] -> Detect Decrease/1
  NOT1/1 -> AND1/2
  SR_Latch/1 -> NOT1/1
  [INPUT] -> AND1/1
  AND1/1 -> DelayEnable_SHORT_PRESS1/1
  [Long_press_falling_edge] -> SR_Latch/1
  [INPUT] -> AND/1
  AND/1 -> DelayEnable_LONG_PRESS1/1
  NOT/1 -> AND/2
  Delay/1 -> NOT/1
  [Long_press_falling_edge] -> Delay/1
  INPUT/1 -> [INPUT]
  task_time_s/1 -> [task_time_s]
  DelayEnable_LONG_PRESS1/1 -> [Long_press_falling_edge]
  Switch3/1 -> Switch/3
  DelayEnable_SHORT_PRESS1/1 -> Detect Decrease4/1
  Constant3/1 -> DelayEnable_LONG_PRESS1/2
  Constant2/1 -> DelayEnable_SHORT_PRESS1/2
  [task_time_s] -> DelayEnable_SHORT_PRESS1/3
  [task_time_s] -> DelayEnable_LONG_PRESS1/3
  Detect Decrease4/1 -> [Short_press_falling_Edge]
  [Long_press_falling_edge] -> Switch/2
  Constant5/1 -> Switch3/1
  Constant4/1 -> Switch/1
  Constant6/1 -> Switch3/3
  Switch/1 -> OUTPUT/1

== system tqd/TQD/TorqueDemand/Signal_convert/Speed Setting Mode/VTQD_SWCSetDownPress_enum ==
  note: Long press or Short press
  INPUT : Inport
  task_time_s : Inport  Port=2
  AND : Logic  AllPortsSameDT=off  OutDataTypeStr=boolean
  AND1 : Logic  AllPortsSameDT=off  OutDataTypeStr=boolean
  Constant1 : Constant  Value=ENUM_SWCBOTTONPRESS_LONGPRESS
  Constant2 : Constant  Value=KTQD_SetSpdShortPLim_s
  Constant3 : Constant  Value=KTQD_SetSpdLongPLim_s
  Constant7 : Constant  Value=ENUM_SWCBOTTONPRESS_SHORTPRESS
  Constant8 : Constant  Value=ENUM_SWCBOTTONPRESS_NOPRESS
  Delay : Delay  DelayLength=1
  DelayEnable_LONG_PRESS1 : hcu_lib/Basic_Blocks/DelayEnable
  DelayEnable_SHORT_PRESS1 : hcu_lib/Basic_Blocks/DelayEnable
  Detect Decrease : simulink/Logic and Bit Operations/Detect Decrease  vinit=0.0  OutDataTypeStr=boolean
  Detect Decrease4 : simulink/Logic and Bit Operations/Detect Decrease  vinit=0.0  OutDataTypeStr=boolean
  NOT : Logic  Operator=NOT  AllPortsSameDT=off  OutDataTypeStr=boolean
  NOT1 : Logic  Operator=NOT  AllPortsSameDT=off  OutDataTypeStr=boolean
  SR_Latch : hcu_lib/Basic_Blocks/SR_Latch
  Switch : Switch  Criteria=u2 ~= 0
  Switch3 : Switch  Criteria=u2 ~= 0
  OUTPUT : Outport
  wires:
  [Short_press_falling_Edge] -> Switch3/2
  Detect Decrease/1 -> SR_Latch/2
  [INPUT] -> Detect Decrease/1
  NOT1/1 -> AND1/2
  SR_Latch/1 -> NOT1/1
  [INPUT] -> AND1/1
  AND1/1 -> DelayEnable_SHORT_PRESS1/1
  [Long_press_falling_edge] -> SR_Latch/1
  [INPUT] -> AND/1
  AND/1 -> DelayEnable_LONG_PRESS1/1
  NOT/1 -> AND/2
  Delay/1 -> NOT/1
  [Long_press_falling_edge] -> Delay/1
  INPUT/1 -> [INPUT]
  task_time_s/1 -> [task_time_s]
  DelayEnable_LONG_PRESS1/1 -> [Long_press_falling_edge]
  Switch3/1 -> Switch/3
  DelayEnable_SHORT_PRESS1/1 -> Detect Decrease4/1
  Constant3/1 -> DelayEnable_LONG_PRESS1/2
  Constant2/1 -> DelayEnable_SHORT_PRESS1/2
  [task_time_s] -> DelayEnable_SHORT_PRESS1/3
  [task_time_s] -> DelayEnable_LONG_PRESS1/3
  Detect Decrease4/1 -> [Short_press_falling_Edge]
  [Long_press_falling_edge] -> Switch/2
  Constant7/1 -> Switch3/1
  Constant1/1 -> Switch/1
  Constant8/1 -> Switch3/3
  Switch/1 -> OUTPUT/1

== system tqd/TQD/TorqueDemand/Signal_convert/VehWeightEst/Calaulation ==
  task_time_s : Inport
  VTQD_VehWeightEstEn_flg : Inport  Port=2
  VTQD_VehWeightEstDis_flg : Inport  Port=3
  VTQD_VehWeightEstEnd_flg : Inport  Port=4
  VVMC_LongAcc_Gps : Inport  Port=5
  VINP_FrEDURealTMTq_Nm : Inport  Port=6
  VINP_RrEDURealTMTq_Nm : Inport  Port=7
  VINP_VehSpeed_kph : Inport  Port=8
  Front Wheel Torque : Subsystem
  Long Acc : Subsystem
  Rear Wheel Torque : Subsystem
  Vehicle Weight : Subsystem
  VTQD_EstLongAccCheckPass_flg : Outport
  VTQD_EstFrRealTqCheckPass_flg : Outport  Port=2
  VTQD_EstRrRealTqCheckPass_flg : Outport  Port=3
  VTQD_EstVehWeight_kg : Outport  Port=4
  wires:
  task_time_s/1 -> [task_time_s]
  VTQD_VehWeightEstEn_flg/1 -> [VTQD_VehWeightEstEn_flg]
  [VVMC_LongAcc_Gps] -> Long Acc/1(VVMC_LongAcc_Gps)
  [VTQD_VehWeightEstEn_flg] -> Long Acc/2(VTQD_VehWeightEstEn_flg)
  [VTQD_VehWeightEstDis_flg] -> Long Acc/3(VTQD_VehWeightEstDis_flg)
  [VTQD_VehWeightEstEnd_flg] -> Long Acc/4(VTQD_VehWeightEstEnd_flg)
  [task_time_s] -> Long Acc/5(task_time_s)
  [VINP_FrEDURealTMTq_Nm] -> Front Wheel Torque/1(VINP_FrEDURealTMTq_Nm)
  [VTQD_VehWeightEstEn_flg] -> Front Wheel Torque/2(VTQD_VehWeightEstEn_flg)
  [VTQD_VehWeightEstDis_flg] -> Front Wheel Torque/3(VTQD_VehWeightEstDis_flg)
  [VTQD_VehWeightEstEnd_flg] -> Front Wheel Torque/4(VTQD_VehWeightEstEnd_flg)
  [task_time_s] -> Front Wheel Torque/5(task_time_s)
  [VINP_RrEDURealTMTq_Nm] -> Rear Wheel Torque/1(VINP_RrEDURealTMTq_Nm)
  [VTQD_VehWeightEstEn_flg] -> Rear Wheel Torque/2(VTQD_VehWeightEstEn_flg)
  [VTQD_VehWeightEstDis_flg] -> Rear Wheel Torque/3(VTQD_VehWeightEstDis_flg)
  [VTQD_VehWeightEstEnd_flg] -> Rear Wheel Torque/4(VTQD_VehWeightEstEnd_flg)
  [task_time_s] -> Rear Wheel Torque/5(task_time_s)
  VTQD_VehWeightEstDis_flg/1 -> [VTQD_VehWeightEstDis_flg]
  VTQD_VehWeightEstEnd_flg/1 -> [VTQD_VehWeightEstEnd_flg]
  VVMC_LongAcc_Gps/1 -> [VVMC_LongAcc_Gps]
  VINP_FrEDURealTMTq_Nm/1 -> [VINP_FrEDURealTMTq_Nm]
  VINP_RrEDURealTMTq_Nm/1 -> [VINP_RrEDURealTMTq_Nm]
  Long Acc/1(VTQD_EstLongAccAvg_Gps) -> [VTQD_EstLongAccAvg_Gps]
  Long Acc/2(VTQD_EstLongAccCheckPass_flg) -> [VTQD_EstLongAccCheckPass_flg]
  Front Wheel Torque/1(VTQD_EstFrRealTqAvg_Nm) -> [VTQD_EstFrRealTqAvg_Nm]
  Front Wheel Torque/2(VTQD_EstFrRealTqCheckPass_flg) -> [VTQD_EstFrRealTqCheckPass_flg]
  Rear Wheel Torque/1(VTQD_EstRrRealTqAvg_Nm) -> [VTQD_EstRrRealTqAvg_Nm]
  Rear Wheel Torque/2(VTQD_EstRrRealTqCheckPass_flg) -> [VTQD_EstRrRealTqCheckPass_flg]
  [VTQD_EstLongAccCheckPass_flg] -> VTQD_EstLongAccCheckPass_flg/1
  [VTQD_EstRrRealTqCheckPass_flg] -> VTQD_EstRrRealTqCheckPass_flg/1
  [VTQD_EstFrRealTqCheckPass_flg] -> VTQD_EstFrRealTqCheckPass_flg/1
  [VTQD_EstFrRealTqAvg_Nm] -> Vehicle Weight/1(VTQD_EstFrRealTqAvg_Nm)
  [VTQD_EstRrRealTqAvg_Nm] -> Vehicle Weight/2(VTQD_EstRrRealTqAvg_Nm)
  [VTQD_EstLongAccAvg_Gps] -> Vehicle Weight/3(VTQD_EstLongAccAvg_Gps)
  [VINP_VehSpeed_kph] -> Vehicle Weight/4(VINP_VehSpeed_kph)
  VINP_VehSpeed_kph/1 -> [VINP_VehSpeed_kph]
  Vehicle Weight/1(VTQD_EstVehWeight_kg) -> [VTQD_EstVehWeight_kg]
  [VTQD_EstVehWeight_kg] -> VTQD_EstVehWeight_kg/1

== system tqd/TQD/TorqueDemand/Signal_convert/VehWeightEst/Condition ==
  VTQD_AfterAvailableTqDemRr_Nm : Inport
  VTQR_NoABSREDUWhlTqReq_Nm : Inport  Port=2
  VTQR_NoABSFEDUWhlTqReq_Nm : Inport  Port=3
  VTQD_AfterAvailableTqDemFr_Nm : Inport  Port=4
  VTQD_GearActualPosn_enum : Inport  Port=5
  VINP_VehSpeed_kph : Inport  Port=6
  VTQD_RollRegenDisableReq_flg : Inport  Port=7
  VINP_RegenMode_enum : Inport  Port=8
  VTQD_LowIdleAccPedal_flg : Inport  Port=9
  VTQD_BrkSwSta_flg : Inport  Port=10
  VINP_RrRBCActive_flg : Inport  Port=11
  VINP_FrRBCActive_flg : Inport  Port=12
  VINP_GRADE_Deg : Inport  Port=13
  task_time_s : Inport  Port=14
  VTQD_VehWeightEstEnd_flg : Inport  Port=15
  AND1 : Logic  Inputs=13  AllPortsSameDT=off  OutDataTypeStr=boolean
  Abs : Abs
  Abs1 : Abs
  Abs2 : Abs
  Add : Sum  Inputs=+-
  Add1 : Sum  Inputs=+-
  Constant1 : Constant  Value=KTQD_VehWeightEstSpdEnLow_kph
  Constant10 : Constant  Value=eps
  Constant11 : Constant  Value=KTQD_VehWeightEstSpdEnUp_kph
  Constant2 : Constant  Value=ENUM_REGENLEVEL_LV1
  Constant3 : Constant  Value=KTQD_RrTqDeviation_Nm
  Constant4 : Constant  Value=KTQD_FrTqDeviation_Nm
  Constant5 : Constant  Value=KTQD_VehWeightEstGradeEn_Deg
  Constant6 : Constant  Value=KTQD_VehWeighEstTime_s
  Constant7 : Constant  Value=KTQD_EstDelayEnTime_s
  Constant8 : Constant  Value=KTQD_EstWeighResetTime_s
  Constant9 : Constant  Value=ENUM_GEARACTUALPOSN_D
  Delay{,1..5} (6 alike) : Delay  DelayLength=1
  DelayEnable : hcu_lib/Basic_Blocks/DelayEnable
  Detect Increase : simulink/Logic and Bit Operations/Detect Increase  vinit=0.0  OutDataTypeStr=boolean
  Equal : RelationalOperator  Operator=<  OutDataTypeStr=boolean  RndMeth=Simplest
  Equal1 : RelationalOperator  Operator===  OutDataTypeStr=boolean  RndMeth=Simplest
  Equal2 : RelationalOperator  Operator=~=  OutDataTypeStr=boolean  RndMeth=Simplest
  Less Than1 : RelationalOperator  Operator=<  OutDataTypeStr=boolean  RndMeth=Simplest
  Less Than2 : RelationalOperator  Operator=>  OutDataTypeStr=boolean  RndMeth=Simplest
  Less Than3 : RelationalOperator  Operator=<=  OutDataTypeStr=boolean  RndMeth=Simplest
  Less Than4 : RelationalOperator  Operator=<=  OutDataTypeStr=boolean  RndMeth=Simplest
  Less Than5 : RelationalOperator  Operator=<=  OutDataTypeStr=boolean  RndMeth=Simplest
  NOT{,1..5} (6 alike) : Logic  Operator=NOT  AllPortsSameDT=off  OutDataTypeStr=boolean
  Relational Operator : RelationalOperator  OutDataTypeStr=boolean  RndMeth=Simplest
  Relational Operator1 : RelationalOperator  OutDataTypeStr=boolean  RndMeth=Simplest
  SR_Latch : hcu_lib/Basic_Blocks/SR_Latch
  Timer : hcu_lib/Basic_Blocks/Timer
  Timer1 : hcu_lib/Basic_Blocks/Timer
  VTQD_VehWeightEstEn_flg : Outport
  VTQD_VehWeightEstDis_flg : Outport  Port=2
  wires:
  Constant9/1 -> Equal1/2
  Less Than1/1 -> AND1/2  "VTQD_VehWeightEstEnCon2_flg"
  Abs/1 -> [VTQD_RrTqErr_Nm]  "VTQD_RrTqErr_Nm"
  Equal1/1 -> AND1/1  "VTQD_VehWeightEstEnCon1_flg"
  Constant11/1 -> Less Than1/2
  [VTQR_NoABSFEDUWhlTqReq_Nm] -> Delay1/1
  Constant4/1 -> Less Than4/2
  Add1/1 -> Abs1/1
  [VTQD_RollRegenDisableReq_flg] -> NOT/1
  [VTQD_RrTqErr_Nm] -> Less Than3/1
  Add/1 -> Abs/1
  [VTQD_BrkSwSta_flg] -> NOT3/1
  [VTQD_FrTqErr_Nm] -> Less Than4/1
  Abs1/1 -> [VTQD_FrTqErr_Nm]  "VTQD_FrTqErr_Nm"
  [VTQD_GearActualPosn_enum] -> Equal1/1
  [VINP_VehSpeed_kph] -> Less Than1/1
  [VINP_RegenMode_enum] -> Equal2/1
  [VTQD_AfterAvailableTqDemFr_Nm] -> Delay4/1
  Constant1/1 -> Less Than2/2
  [VTQD_AfterAvailableTqDemRr_Nm] -> Delay2/1
  Less Than4/1 -> AND1/8  "VTQD_VehWeightEstEnCon7_flg"
  [VINP_RrRBCActive_flg] -> NOT4/1
  [VTQR_NoABSREDUWhlTqReq_Nm] -> Delay3/1
  NOT/1 -> AND1/4  "VTQD_VehWeightEstEnCon4_flg"
  [VINP_FrRBCActive_flg] -> NOT5/1
  Constant5/1 -> Less Than5/2
  Equal2/1 -> AND1/5  "VTQD_VehWeightEstEnCon5_flg"
  [VTQD_LowIdleAccPedal_flg] -> AND1/6
  Constant2/1 -> Equal2/2
  Less Than3/1 -> AND1/7  "VTQD_VehWeightEstEnCon6_flg"
  Less Than2/1 -> AND1/3  "VTQD_VehWeightEstEnCon3_flg"
  [VINP_VehSpeed_kph] -> Less Than2/1
  Less Than5/1 -> AND1/12  "VTQD_VehWeightEstEnCon11_flg"
  [VINP_GRADE_Deg] -> Abs2/1
  Abs2/1 -> Less Than5/1
  Constant3/1 -> Less Than3/2
  VTQD_AfterAvailableTqDemRr_Nm/1 -> [VTQD_AfterAvailableTqDemRr_Nm]
  VTQR_NoABSREDUWhlTqReq_Nm/1 -> [VTQR_NoABSREDUWhlTqReq_Nm]
  VTQD_AfterAvailableTqDemFr_Nm/1 -> [VTQD_AfterAvailableTqDemFr_Nm]
  VTQR_NoABSFEDUWhlTqReq_Nm/1 -> [VTQR_NoABSFEDUWhlTqReq_Nm]
  VTQD_GearActualPosn_enum/1 -> [VTQD_GearActualPosn_enum]
  VINP_VehSpeed_kph/1 -> [VINP_VehSpeed_kph]
  VTQD_RollRegenDisableReq_flg/1 -> [VTQD_RollRegenDisableReq_flg]
  VINP_RegenMode_enum/1 -> [VINP_RegenMode_enum]
  VTQD_LowIdleAccPedal_flg/1 -> [VTQD_LowIdleAccPedal_flg]
  VTQD_BrkSwSta_flg/1 -> [VTQD_BrkSwSta_flg]
  VINP_RrRBCActive_flg/1 -> [VINP_RrRBCActive_flg]
  VINP_FrRBCActive_flg/1 -> [VINP_FrRBCActive_flg]
  VINP_GRADE_Deg/1 -> [VINP_GRADE_Deg]
  [VTQD_VehWeightEstEn_flg] -> VTQD_VehWeightEstEn_flg/1
  Relational Operator/1 -> [VTQD_VehWeightEstDis_flg]  "VTQD_VehWeightEstDis_flg"
  Timer/1 -> Relational Operator/1
  NOT1/1 -> Timer/2
  [VTQD_VehWeightEstEn_flg] -> NOT1/1, Timer/1
  Constant6/1 -> Relational Operator/2, Timer/4
  [VTQD_VehWeightEstDis_flg] -> VTQD_VehWeightEstDis_flg/1
  task_time_s/1 -> [task_time_s]
  AND1/1 -> DelayEnable/1
  DelayEnable/1 -> [VTQD_VehWeightEstEn_flg]  "VTQD_VehWeightEstEn_flg"
  [task_time_s] -> DelayEnable/3
  Constant7/1 -> DelayEnable/2
  [VTQD_VehWeightEstEnd_flg] -> Detect Increase/1
  Detect Increase/1 -> SR_Latch/1
  SR_Latch/1 -> NOT2/1, Timer1/1
  NOT2/1 -> Timer1/2
  Constant8/1 -> Relational Operator1/2, Timer1/4
  Timer1/1 -> [VTQD_EstVehWeightResetTime_s], Relational Operator1/1  "VTQD_EstVehWeightResetTime_s"
  Relational Operator1/1 -> [VTQD_EstVehWeitResetFinish_flg]  "VTQD_EstVehWeitResetFinish_flg"
  [VTQD_EstVehWeitResetFinish_flg] -> Delay/1
  Delay/1 -> SR_Latch/2
  [VTQD_EstVehWeightResetTime_s] -> Delay5/1
  Constant10/1 -> Equal/2
  Equal/1 -> AND1/13  "VTQD_VehWeightEstEnCon12_flg"
  VTQD_VehWeightEstEnd_flg/1 -> [VTQD_VehWeightEstEnd_flg]
  Delay1/1 -> Add1/1
  Delay2/1 -> Add/1
  Delay3/1 -> Add/2
  Delay4/1 -> Add1/2
  Delay5/1 -> Equal/1
  NOT3/1 -> AND1/9  "VTQD_VehWeightEstEnCon8_flg"
  NOT4/1 -> AND1/10  "VTQD_VehWeightEstEnCon9_flg"
  NOT5/1 -> AND1/11  "VTQD_VehWeightEstEnCon10_flg"
  [task_time_s] -> Timer/3
  [task_time_s] -> Timer1/3

== system tqd/TQD/TorqueDemand/Signal_convert/VehWeightEst/Desicion ==
  task_time_s : Inport
  VTQD_VehWeightEstDis_flg : Inport  Port=2
  VTQD_EstVehWeight_kg : Inport  Port=3
  VINP_DriverSeatBeltCmd_flg : Inport  Port=4
  VINP_PsngrSeatBeltCmd_flg : Inport  Port=5
  VINP_RDriverSeatBeltCmd_flg : Inport  Port=6
  VINP_RCenterSeatBeltCmd_flg : Inport  Port=7
  VINP_RPsngrSeatBeltCmd_flg : Inport  Port=8
  VTQD_EstLongAccCheckPass_flg : Inport  Port=9
  VTQD_EstFrRealTqCheckPass_flg : Inport  Port=10
  VTQD_EstRrRealTqCheckPass_flg : Inport  Port=11
  AND : Logic  Inputs=5  AllPortsSameDT=off  OutDataTypeStr=boolean
  Add : Sum  Inputs=+++++
  Constant1 : Constant  Value=eps
  Constant{2,4,6,8,10} (5 alike) : Constant  Value=ZERO_INT
  Constant{3,5,7,9,11} (5 alike) : Constant  Value=ONE_INT
  Constant12 : Constant  Value=KTQD_EstEndDelayTime_s
  Data Type Conversion : DataTypeConversion  OutDataTypeStr=single
  Delay : Delay  DelayLength=1
  Delay1 : Delay  DelayLength=1
  DelayEnable : hcu_lib/Basic_Blocks/DelayEnable
  Equal : RelationalOperator  OutDataTypeStr=boolean  RndMeth=Simplest
  MTQD_EstInitVehWeight_Y_kg : Lookup_n-D  NumberOfTableDimensions=1  BreakpointsForDimension1=ATQD_EstInitVehWeight_X_c  Table=MTQD_EstInitVehWeight_Y_kg  ExtrapMethod=Clip  InternalRulePriority=Speed  RndMeth=Simplest  InputSameDT=on
  NOT : Logic  Operator=NOT  AllPortsSameDT=off  OutDataTypeStr=boolean
  Switch{,1..6} (7 alike) : Switch  Criteria=u2 > Threshold
  VTQD_VehWeightEstEnd_flg : Outport
  VTQD_EstVehWeightResult_kg : Outport  Port=2
  wires:
  Constant7/1 -> Switch4/1
  Constant1/1 -> Equal/2
  Switch2/1 -> Add/1
  [VINP_DriverSeatBeltCmd_flg] -> Switch2/2
  [VINP_RCenterSeatBeltCmd_flg] -> Switch4/2
  Switch5/1 -> Add/4
  Equal/1 -> Switch1/2
  Constant10/1 -> Switch6/3
  [VTQD_VehWeightEstDis_flg] -> AND/1
  Switch6/1 -> Add/5
  Delay/1 -> NOT/1
  Switch3/1 -> Add/2
  Constant6/1 -> Switch4/3
  Constant3/1 -> Switch2/1
  [VTQD_EstActVehWeight_kg] -> Switch1/1
  Constant2/1 -> Switch2/3
  [VTQD_VehWeightEstEnter_flg] -> Switch/2
  Constant11/1 -> Switch6/1
  Switch1/1 -> [VTQD_EstVehWeightResult_kg]  "VTQD_EstVehWeightResult_kg"
  Constant4/1 -> Switch3/3
  Constant5/1 -> Switch3/1
  [VINP_RDriverSeatBeltCmd_flg] -> Switch5/2
  Switch/1 -> Delay1/1, [VTQD_EstActVehWeight_kg]  "VTQD_EstActVehWeight_kg"
  AND/1 -> [VTQD_VehWeightEstEnter_flg]  "VTQD_VehWeightEstEnter_flg"
  [VINP_RPsngrSeatBeltCmd_flg] -> Switch6/2
  [VTQD_EstActVehWeight_kg] -> Equal/1
  [VINP_PsngrSeatBeltCmd_flg] -> Switch3/2
  Delay1/1 -> Switch/3
  [VTQD_EstInitVehWeight_kg] -> Switch1/3
  Constant9/1 -> Switch5/1
  Constant8/1 -> Switch5/3
  [VTQD_EstVehWeight_kg] -> Switch/1
  [VTQD_VehWeightEstEnd_flg] -> Delay/1
  NOT/1 -> AND/2
  Switch4/1 -> Add/3
  [VTQD_VehWeightEstDis_flg] -> DelayEnable/1
  Constant12/1 -> DelayEnable/2
  [task_time_s] -> DelayEnable/3
  DelayEnable/1 -> [VTQD_VehWeightEstEnd_flg]  "VTQD_VehWeightEstEnd_flg"
  task_time_s/1 -> [task_time_s]
  [VTQD_VehWeightEstEnd_flg] -> VTQD_VehWeightEstEnd_flg/1
  VTQD_VehWeightEstDis_flg/1 -> [VTQD_VehWeightEstDis_flg]
  VTQD_EstVehWeight_kg/1 -> [VTQD_EstVehWeight_kg]
  [VTQD_EstVehWeightResult_kg] -> VTQD_EstVehWeightResult_kg/1
  VINP_DriverSeatBeltCmd_flg/1 -> [VINP_DriverSeatBeltCmd_flg]
  VINP_PsngrSeatBeltCmd_flg/1 -> [VINP_PsngrSeatBeltCmd_flg]
  VINP_RDriverSeatBeltCmd_flg/1 -> [VINP_RDriverSeatBeltCmd_flg]
  VINP_RCenterSeatBeltCmd_flg/1 -> [VINP_RCenterSeatBeltCmd_flg]
  VINP_RPsngrSeatBeltCmd_flg/1 -> [VINP_RPsngrSeatBeltCmd_flg]
  VTQD_EstRrRealTqCheckPass_flg/1 -> [VTQD_EstRrRealTqCheckPass_flg]
  VTQD_EstFrRealTqCheckPass_flg/1 -> [VTQD_EstFrRealTqCheckPass_flg]
  VTQD_EstLongAccCheckPass_flg/1 -> [VTQD_EstLongAccCheckPass_flg]
  [VTQD_EstLongAccCheckPass_flg] -> AND/3
  [VTQD_EstFrRealTqCheckPass_flg] -> AND/4
  [VTQD_EstRrRealTqCheckPass_flg] -> AND/5
  MTQD_EstInitVehWeight_Y_kg/1 -> [VTQD_EstInitVehWeight_kg]  "VTQD_EstInitVehWeight_kg"
  Data Type Conversion/1 -> MTQD_EstInitVehWeight_Y_kg/1
  Add/1 -> Data Type Conversion/1  "VTQD_EstInitVehWightX_c"
